simulink model "zad6_sim"  (R2014b)
settings: Solver=ode45  StartTime=0.0  StopTime=10  RelTol=1e-3
values from neighbouring files (symbols this model uses):
  K = acker(A,B, poles(i,:))    [zad10.m]    (also in zad6.m = acker(A,B, poles(i,:)'); zad9.m = acker(A,B, [0.2 0.5+0.1j 0.5-0.1j]))
  Tp = 0.25    [setparam.m]    (also in zad1.m)
  x1_ini = 0.0    (= 0)    [setparam.m]    (also in zad10.m = 1; zad4.m; zad6.m = 1; zad9.m = 1)
  x2_ini = 0.0    (= 0)    [setparam.m]    (also in zad10.m = -5; zad4.m; zad6.m = -5; zad9.m = -5)
  x3_ini = 0.0    (= 0)    [setparam.m]    (also in zad10.m = 1; zad4.m = 1; zad6.m = 1; zad9.m = 1)
settings Model: Creator=kuba  LastModifiedBy=kuba
settings DebuggingCC: SolverPrmCheckMsg=none

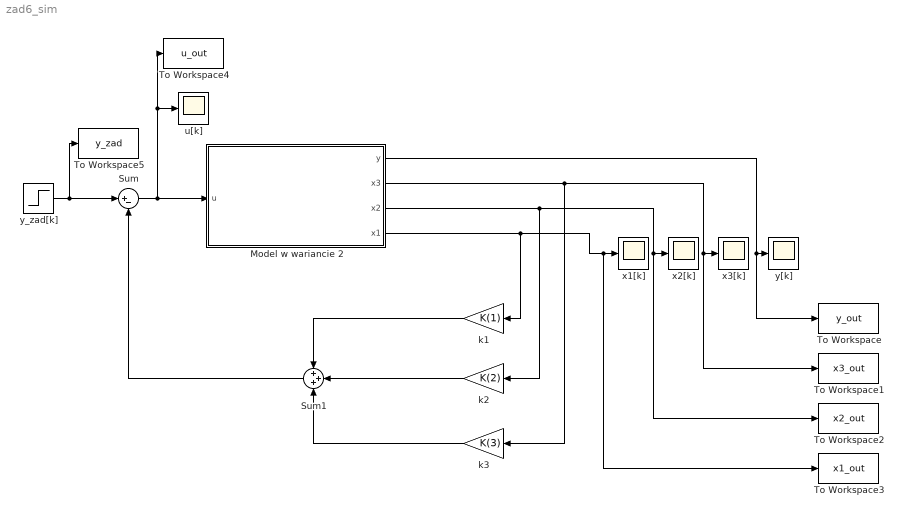
== system zad6_sim ==
  "Model w wariancie 2 " : Subsystem
  Sum : Sum  Inputs=|+-
  Sum1 : Sum  Inputs=+++
  To Workspace : ToWorkspace  VariableName=y_out  SaveFormat=Timeseries  SampleTime=-1
  To Workspace1 : ToWorkspace  VariableName=x3_out  SaveFormat=Timeseries  SampleTime=-1
  To Workspace2 : ToWorkspace  VariableName=x2_out  SaveFormat=Timeseries  SampleTime=-1
  To Workspace3 : ToWorkspace  VariableName=x1_out  SaveFormat=Timeseries  SampleTime=-1
  To Workspace4 : ToWorkspace  VariableName=u_out  SaveFormat=Timeseries  SampleTime=-1
  To Workspace5 : ToWorkspace  VariableName=y_zad  SaveFormat=Timeseries  SampleTime=-1
  k1 : Gain  Gain=K(1)
  k2 : Gain  Gain=K(2)
  "k3 " : Gain  Gain=K(3)
  u[k] : Scope
      settings: SaveName=ScopeData4
  x1[k] : Scope
  x2[k] : Scope
      settings: SaveName=ScopeData2
  x3[k] : Scope
      settings: SaveName=ScopeData3
  y[k] : Scope
  y_zad[k] : Step  After=0  SampleTime=0
  wires:
  "Model w wariancie 2 "/1(y) -> y[k]/1, To Workspace/1
  "Model w wariancie 2 "/4(x1) -> k1/1, To Workspace3/1, x1[k]/1
  "Model w wariancie 2 "/2(x3) -> "k3 "/1, To Workspace1/1, x3[k]/1
  y_zad[k]/1 -> To Workspace5/1, Sum/1
  Sum1/1 -> Sum/2
  k2/1 -> Sum1/2
  k1/1 -> Sum1/1
  "k3 "/1 -> Sum1/3
  Sum/1 -> To Workspace4/1, u[k]/1, "Model w wariancie 2 "/1(u)
  "Model w wariancie 2 "/3(x2) -> k2/1, To Workspace2/1, x2[k]/1

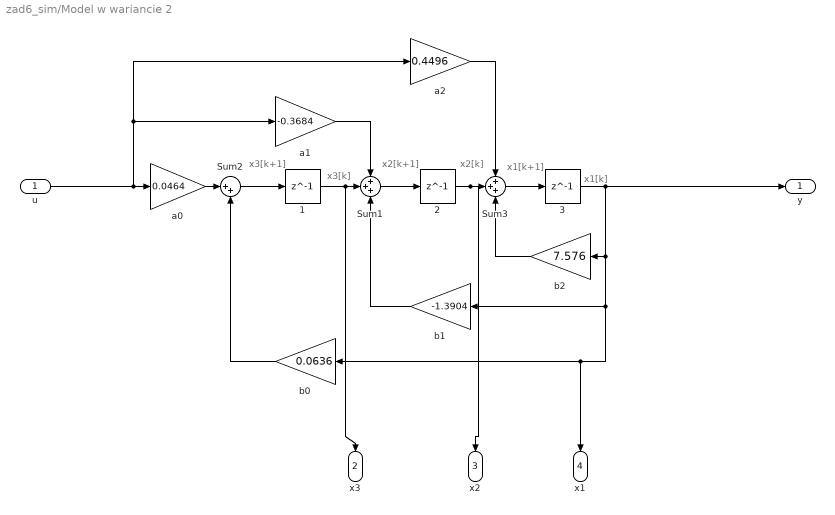
== system zad6_sim/Model w wariancie 2  ==
  note: x3[k]
  note: x3[k+1]
  note: x2[k]
  note: x2[k+1]
  note: x1[k]
  note: x1[k+1]
  u : Inport
  1 : Delay  DelayLength=1  InitialCondition=x1_ini  SampleTime=Tp
  2 : Delay  DelayLength=1  InitialCondition=x2_ini  SampleTime=Tp
  3 : Delay  DelayLength=1  InitialCondition=x3_ini  SampleTime=Tp
  Sum1 : Sum  Inputs=+++
  Sum2 : Sum  Inputs=|++
  Sum3 : Sum  Inputs=+++
  "a0 " : Gain  Gain=0.0464
  a1 : Gain  Gain=-0.3684
  a2 : Gain  Gain=0.4496
  "b0 " : Gain  Gain=0.0636
  b1 : Gain  Gain=-1.3904
  b2 : Gain  Gain=7.576
  y : Outport
  x3 : Outport  Port=2
  x2 : Outport  Port=3
  x1 : Outport  Port=4
  wires:
  2/1 -> x2/1, Sum3/2
  b1/1 -> Sum1/3
  "a0 "/1 -> Sum2/1
  Sum1/1 -> 2/1
  3/1 -> y/1, "b0 "/1, x1/1, b1/1, b2/1
  a1/1 -> Sum1/1
  a2/1 -> Sum3/1
  1/1 -> x3/1, Sum1/2
  Sum3/1 -> 3/1
  Sum2/1 -> 1/1
  b2/1 -> Sum3/3
  u/1 -> a2/1, a1/1, "a0 "/1
  "b0 "/1 -> Sum2/2
